simulink model "microgrid"  (R2021b)
settings: Solver=ode23tb  StartTime=0.0  StopTime=1  FixedStep=5e-6  RelTol=1e-3  EnableMultiTasking=on
PreLoadFcn:
  | % ---- microgrid : PreLoadFcn -------------------------------------
  | % Loads every base-workspace parameter this model needs.
  | %   SolarPVMPPTBoostData.mlx : PV array, boost converter, MPPT controller
  | %   microgridParams.m        : bus, battery, grid, drain, droop  (struct mg)
  | try
  |     mgDir = fileparts(which('microgrid'));
  |     if ~isempty(mgDir) && ~contains([path pathsep], [mgDir pathsep])
  |         addpath(mgDir);
  |     end
  |     evalc('SolarPVMPPTBoostData');
  |     microgridParams;
  |     clear mgDir
  |     disp('microgrid: parameters loaded (SolarPVMPPTBoostData + microgridParams).');
  | catch mgErr
  |     warning('microgrid:paramLoadFailed', ...
  |             'Could not load model parameters: %s', mgErr.message);
  |     clear mgErr
  | end
values from neighbouring files (symbols this model uses):
  mg = evalin('base','mg')    [microgridCheck.m]    (also in microgridParams.m = struct(); microgridScenario.m)
undefined symbols (not defined in the file or in its folder): boostController, dcVoltage, Ion, Lithium, sensor, solarPanel, solarPlant
libraries: powerlib_extras x46, fl_lib x12, simulink x8, nesl_utility x8, spsSeriesRLCBranchLib x7, spsCurrentMeasurementLib x7, spsGroundLib x6, spsVoltageMeasurementLib x6, spsIGBTDiodeLib x4, spsVariableResistorLib x4, slpidlib x4, ee_lib x3
(part 3 of 3)

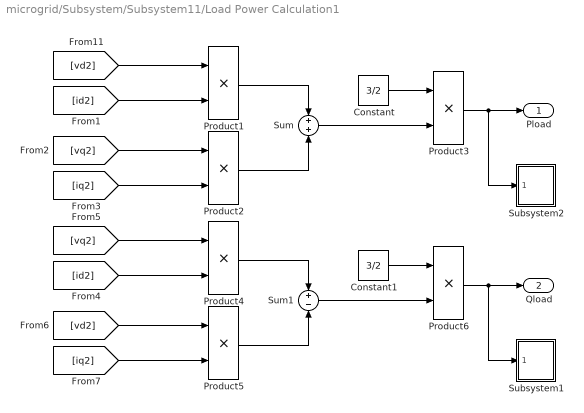
== system microgrid/Subsystem/Subsystem11/Load Power Calculation1 ==
  Constant : Constant  Value=3/2
  Constant1 : Constant  Value=3/2
  Product{1..6} (6 alike) : Product  RndMeth=Zero
  Subsystem1 : Subsystem
  Subsystem2 : Subsystem
  Sum : Sum  Inputs=+|+
  Sum1 : Sum  Inputs=+|-
  Pload : Outport
  Qload : Outport  Port=2
  wires:
  Product6/1 -> Qload/1, Subsystem1/1(Qacload)
  Constant1/1 -> Product6/1
  Sum1/1 -> Product6/2
  Product5/1 -> Sum1/2
  Product4/1 -> Sum1/1
  [iq2] -> Product5/2
  [vd2] -> Product5/1
  [id2] -> Product4/2
  [vq2] -> Product4/1
  Product3/1 -> Pload/1, Subsystem2/1(Pload)
  Constant/1 -> Product3/1
  Sum/1 -> Product3/2
  Product2/1 -> Sum/2
  Product1/1 -> Sum/1
  [iq2] -> Product2/2
  [vq2] -> Product2/1
  [id2] -> Product1/2
  [vd2] -> Product1/1

== system microgrid/Subsystem/Subsystem11/Load Power Calculation2 ==
  Constant : Constant  Value=3/2
  Constant1 : Constant  Value=3/2
  Product{1..6} (6 alike) : Product  RndMeth=Zero
  Subsystem1 : Subsystem
  Subsystem2 : Subsystem
  Sum : Sum  Inputs=+|+
  Sum1 : Sum  Inputs=+|-
  Pload : Outport
  Qload : Outport  Port=2
  wires:
  [vd3] -> Product1/1
  [id3] -> Product1/2
  [vq3] -> Product2/1
  [iq3] -> Product2/2
  Product1/1 -> Sum/1
  Product2/1 -> Sum/2
  Sum/1 -> Product3/2
  Constant/1 -> Product3/1
  Product3/1 -> Pload/1, Subsystem2/1(Pload)
  [vq3] -> Product4/1
  [id3] -> Product4/2
  [vd3] -> Product5/1
  [iq3] -> Product5/2
  Product4/1 -> Sum1/1
  Product5/1 -> Sum1/2
  Sum1/1 -> Product6/2
  Constant1/1 -> Product6/1
  Product6/1 -> Qload/1, Subsystem1/1(Qacload)

== system microgrid/PV + Boost/PV Control/Constant Voltage/Current control ==
  e : Inport
  Integrator : Integrator  LimitOutput=on  UpperSaturationLimit=1.5  LowerSaturationLimit=-1.5
  Ki : Gain  Gain=1/boostController.mppCurrentZeroTimeConst
  Kp : Gain  Gain=boostController.mppCurrentGain
  Saturation : Saturate  UpperLimit=1.5  LowerLimit=-1.5
  Sum7 : Sum  Inputs=|++
  u : Outport  VectorParamsAs1DForOutWhenUnconnected=off
  wires:
  Integrator/1 -> Sum7/2
  Saturation/1 -> u/1
  Sum7/1 -> Saturation/1
  e/1 -> Kp/1
  Kp/1 -> Ki/1, Sum7/1
  Ki/1 -> Integrator/1

== system microgrid/PV + Boost/PV Control/Constant Voltage/Voltage control ==
  e : Inport
  1/T : Gain  Gain=1/boostController.mppVoltageZeroTimeConst
  Integrator : Integrator  LimitOutput=on  UpperSaturationLimit=boostController.mppVoltageLoopMax  LowerSaturationLimit=boostController.mppVoltageLoopMin
  Kp : Gain  Gain=boostController.mppVoltageGain
  Saturation : Saturate  UpperLimit=boostController.mppVoltageLoopMax  LowerLimit=boostController.mppVoltageLoopMin
  Sum7 : Sum  Inputs=|++
  u : Outport  VectorParamsAs1DForOutWhenUnconnected=off
  wires:
  Integrator/1 -> Sum7/2
  Saturation/1 -> u/1
  Sum7/1 -> Saturation/1
  e/1 -> Kp/1
  Kp/1 -> 1/T/1, Sum7/1
  1/T/1 -> Integrator/1

== system microgrid/PV + Boost/PV Control/Maximum Power Point/MPPT ==
  Ipv : Inport
  Vpv : Inport  Port=2
  Add : Sum
  Constant1 : Constant  Value=solarPlant.voltMPPT
  Initialize : Subsystem
  MPPT Algorithm : Subsystem  Variant=on
  MPPT End Value : Constant  Value=solarPlant.endMPPTValue
  Subtract5 : Sum  Inputs=-+
  Switch : Switch  Threshold=solarPlant.endMPPTValue
  Switch5 : Switch  Criteria=u2 > Threshold  Threshold=solarPlant.startMPPTValue
  start MPPT Voltage : Constant  Value=solarPlant.startMPPTValue
  Vmpp : Outport  VectorParamsAs1DForOutWhenUnconnected=off
  tag scope: Ipvnow=global, Vdec=global, Vinc=global, Vpvnow=global
  wires:
  Switch5/1 -> Add/1, Subtract5/2
  Add/1 -> [Vinc]  "INC"
  start MPPT Voltage/1 -> Switch5/3
  Vpv/1 -> [Vpvnow], Switch5/2, Switch5/1, MPPT Algorithm/2(Vpv)
  Constant1/1 -> Add/2, Subtract5/1
  Subtract5/1 -> [Vdec]  "DEC"
  Ipv/1 -> [Ipvnow], MPPT Algorithm/1(Ipv)
  MPPT Algorithm/1(Vmpp) -> Initialize/1(In)
  Initialize/1(Out) -> Switch/3, Switch/2
  Switch/1 -> Vmpp/1
  MPPT End Value/1 -> Switch/1

== system microgrid/PV + Boost/PV Control/Maximum Power Point/MPPT Subsystem ==
  note: Current controller
  note: Voltage Control
  VpvRef : Inport
  Vpv : Inport  Port=2
  IL : Inport  Port=3
  "Vo " : Inport  Port=4
  Constant : Constant  Value=solarPlant.startMPPTValue
  Current control : Subsystem
  Divide : Product  Inputs=*/
  PWM Generator : eePwmGenerator/PWM Generator  CarrCount=Up  Tper=1/solarPlant.converterSwitchingFrequency  Tdelay=0  Ts=1/(10*solarPlant.converterSwitchingFrequency)
  Rate Transition1 : RateTransition  OutPortSampleTime=1/(10*solarPlant.converterSwitchingFrequency)
  Saturation : Saturate  UpperLimit=1  LowerLimit=0
  Subtract : Sum  Inputs=-+
  Sum : Sum  Inputs=|+-
  Sum2 : Sum  Inputs=|--
  Sum3 : Sum  Inputs=|++
  Switch : Switch  Criteria=u2 > Threshold  Threshold=dcVoltage.avgDCVoltage*0.7
  Transfer Fcn (with initial states) : simulink_extras/Additional Linear/Transfer Fcn (with initial states)  N=[1]  D=[0.00001 1]  X0=solarPlant.startMPPTValue
  Voltage control : Subsystem
  G : Outport
  wires:
  Subtract/1 -> Divide/1
  Voltage control/1(u) -> Sum2/1
  Current control/1(u) -> Sum3/1
  Sum2/1 -> Current control/1(e)
  "Vo "/1 -> Switch/2, Switch/1
  VpvRef/1 -> Transfer Fcn (with initial states)/1
  Constant/1 -> Switch/3
  Switch/1 -> Divide/2, Subtract/2
  Vpv/1 -> Subtract/1, Sum/2
  Saturation/1 -> Rate Transition1/1  "set"
  Rate Transition1/1 -> PWM Generator/1
  PWM Generator/1 -> G/1
  Divide/1 -> Sum3/2
  Sum/1 -> Voltage control/1(e)
  IL/1 -> Sum2/2
  Transfer Fcn (with initial states)/1 -> Sum/1
  Sum3/1 -> Saturation/1

== system microgrid/Subsystem/Inverter Control Measurements3/PLL/PI ==
  e : Inport
  Gain1 : Gain  Gain=10
  Gain2 : Gain  Gain=100
  Integrator : Integrator
  Saturation : Saturate  UpperLimit=inf  LowerLimit=-inf
  Sum1 : Sum  Inputs=|++
  w : Outport
  wires:
  Integrator/1 -> Sum1/2
  Gain1/1 -> Sum1/1
  e/1 -> Gain2/1, Gain1/1
  Gain2/1 -> Integrator/1
  Saturation/1 -> w/1
  Sum1/1 -> Saturation/1

== system microgrid/Subsystem/Inverter Control Measurements3/PLL/Subsystem3 ==
  wabc : Inport
  LPF vq7 : powerlib_extras/Discrete  Control Blocks/Discrete 1st-Order Filter  FilterType=Lowpass  Tc=10e-3  Ts=5e-6  Initialize=off  Vac_Init=[0.8 -25 60]  Vdc_Init=0  PlotResponse=off  param1=[1 100 0.1]
      settings: SourceProductBaseCode=PS
  To Workspace1 : ToWorkspace  VariableName=wabc_real  SampleTime=-1
  To Workspace2 : ToWorkspace  VariableName=wabc_real_fil  SampleTime=-1
  Zero-Order Hold : ZeroOrderHold  SampleTime=5e-6
  tag scope: w_abc=global
  wires:
  LPF vq7/1 -> To Workspace2/1
  wabc/1 -> Zero-Order Hold/1
  Zero-Order Hold/1 -> LPF vq7/1, To Workspace1/1, [w_abc]

== system microgrid/Subsystem/Inverter Control Measurements3/PLL/abc  - d//q ==
  abc : Inport
  tita : Inport  Port=2
  abc  - alfa/beta : Subsystem
  alfa/beta - dq : Subsystem
  d/q : Outport
  wires:
  tita/1 -> alfa/beta - dq/2(tita)
  alfa/beta - dq/1(d/q) -> d/q/1
  abc/1 -> abc  - alfa/beta/1(abc)
  abc  - alfa/beta/1(alfa/beta) -> alfa/beta - dq/1(alfa/beta)

== system microgrid/Subsystem/Subsystem11/Load Power Calculation1/Subsystem1 ==
  Qacload : Inport
  LPF vq7 : powerlib_extras/Discrete  Control Blocks/Discrete 1st-Order Filter  FilterType=Lowpass  Tc=10e-3  Ts=5e-6  Initialize=off  Vac_Init=[0.8 -25 60]  Vdc_Init=0  PlotResponse=off  param1=[1 100 0.1]
      settings: SourceProductBaseCode=PS
  To Workspace1 : ToWorkspace  VariableName=Qacload3  SampleTime=-1
  To Workspace2 : ToWorkspace  VariableName=Qacload_3  SampleTime=-1
  Zero-Order Hold : ZeroOrderHold  SampleTime=5e-6
  tag scope: Qacload3=global
  wires:
  Qacload/1 -> Zero-Order Hold/1
  Zero-Order Hold/1 -> [Qacload3], To Workspace2/1, LPF vq7/1
  LPF vq7/1 -> To Workspace1/1

== system microgrid/Subsystem/Subsystem11/Load Power Calculation1/Subsystem2 ==
  Pload : Inport
  LPF vq7 : powerlib_extras/Discrete  Control Blocks/Discrete 1st-Order Filter  FilterType=Lowpass  Tc=10e-3  Ts=5e-6  Initialize=off  Vac_Init=[0.8 -25 60]  Vdc_Init=0  PlotResponse=off  param1=[1 100 0.1]
      settings: SourceProductBaseCode=PS
  To Workspace1 : ToWorkspace  VariableName=Pacload3  SampleTime=-1
  To Workspace2 : ToWorkspace  VariableName=Pacload_3  SampleTime=-1
  Zero-Order Hold : ZeroOrderHold  SampleTime=5e-6
  tag scope: Pacload3=global
  wires:
  Pload/1 -> Zero-Order Hold/1
  Zero-Order Hold/1 -> [Pacload3], To Workspace2/1, LPF vq7/1
  LPF vq7/1 -> To Workspace1/1

== system microgrid/Subsystem/Subsystem11/Load Power Calculation2/Subsystem1 ==
  Qacload : Inport
  LPF vq7 : powerlib_extras/Discrete  Control Blocks/Discrete 1st-Order Filter  FilterType=Lowpass  Tc=10e-3  Ts=5e-6  Initialize=off  Vac_Init=[0.8 -25 60]  Vdc_Init=0  PlotResponse=off  param1=[1 100 0.1]
      settings: SourceProductBaseCode=PS
  To Workspace1 : ToWorkspace  VariableName=Qacload2  SampleTime=-1
  To Workspace2 : ToWorkspace  VariableName=Qacload_2  SampleTime=-1
  Zero-Order Hold : ZeroOrderHold  SampleTime=5e-6
  tag scope: Qacload2=global
  wires:
  Qacload/1 -> Zero-Order Hold/1
  Zero-Order Hold/1 -> [Qacload2], To Workspace2/1, LPF vq7/1
  LPF vq7/1 -> To Workspace1/1

== system microgrid/Subsystem/Subsystem11/Load Power Calculation2/Subsystem2 ==
  Pload : Inport
  LPF vq7 : powerlib_extras/Discrete  Control Blocks/Discrete 1st-Order Filter  FilterType=Lowpass  Tc=10e-3  Ts=5e-6  Initialize=off  Vac_Init=[0.8 -25 60]  Vdc_Init=0  PlotResponse=off  param1=[1 100 0.1]
      settings: SourceProductBaseCode=PS
  To Workspace1 : ToWorkspace  VariableName=Pacload2  SampleTime=-1
  To Workspace2 : ToWorkspace  VariableName=Pacload_2  SampleTime=-1
  Zero-Order Hold : ZeroOrderHold  SampleTime=5e-6
  tag scope: Pacload2=global
  wires:
  Pload/1 -> Zero-Order Hold/1
  Zero-Order Hold/1 -> [Pacload2], To Workspace2/1, LPF vq7/1
  LPF vq7/1 -> To Workspace1/1

== system microgrid/PV + Boost/PV Control/Maximum Power Point/MPPT/Initialize ==
  In : Inport
  Constant : Constant  Value=solarPlant.startMPPTValue
  Constant2 : Constant
  Integrator : Integrator
  Switch1 : Switch  Criteria=u2 > Threshold  Threshold=solarPlant.startMPPTValue
  Switch2 : Switch  Criteria=u2 > Threshold  Threshold=solarPlant.timeMPPT
  Out : Outport
  wires:
  Constant/1 -> Switch1/3
  Switch1/1 -> Switch2/1
  In/1 -> Switch1/2, Switch1/1
  Switch2/1 -> Out/1
  Constant2/1 -> Integrator/1
  [Vpvnow] -> Switch2/3
  Integrator/1 -> Switch2/2

== system microgrid/PV + Boost/PV Control/Maximum Power Point/MPPT/MPPT Algorithm ==
  Ipv : Inport
  Vpv : Inport  Port=2
  IncrementalConductance : Subsystem  VariantControl=incrementalConductance
  PerturbationAndObsrvation : Subsystem  VariantControl=perturbationAndObservation
  Vmpp : Outport  VectorParamsAs1DForOutWhenUnconnected=off

== system microgrid/PV + Boost/PV Control/Maximum Power Point/MPPT Subsystem/Current control ==
  e : Inport
  Integrator : Integrator  InitialCondition=1  LimitOutput=on  UpperSaturationLimit=1  LowerSaturationLimit=-0.5
  Ki : Gain  Gain=1/boostController.mppCurrentZeroTimeConst
  Kp : Gain  Gain=boostController.mppCurrentGain
  Saturation : Saturate  UpperLimit=1  LowerLimit=-0.3
  Sum7 : Sum  Inputs=|++
  u : Outport  VectorParamsAs1DForOutWhenUnconnected=off
  wires:
  Integrator/1 -> Sum7/2
  Saturation/1 -> u/1
  Sum7/1 -> Saturation/1
  e/1 -> Kp/1
  Kp/1 -> Ki/1, Sum7/1
  Ki/1 -> Integrator/1

== system microgrid/PV + Boost/PV Control/Maximum Power Point/MPPT Subsystem/Voltage control ==
  e : Inport
  1/T : Gain  Gain=1/boostController.mppVoltageZeroTimeConst
  Integrator : Integrator  LimitOutput=on  UpperSaturationLimit=boostController.mppVoltageLoopMax  LowerSaturationLimit=boostController.mppVoltageLoopMin
  Kp : Gain  Gain=boostController.mppVoltageGain
  Saturation : Saturate  UpperLimit=boostController.mppVoltageLoopMax  LowerLimit=boostController.mppVoltageLoopMin
  Sum7 : Sum  Inputs=|++
  u : Outport  VectorParamsAs1DForOutWhenUnconnected=off
  wires:
  Integrator/1 -> Sum7/2
  Saturation/1 -> u/1
  Sum7/1 -> Saturation/1
  e/1 -> Kp/1
  Kp/1 -> 1/T/1, Sum7/1
  1/T/1 -> Integrator/1

== system microgrid/Subsystem/Inverter Control Measurements3/PLL/abc  - d//q/abc  - alfa//beta ==
  abc : Inport
  Mux : Mux  Inputs=2
  d_s : Fcn  Expr=(-1/sqrt(3)*u[2])+(1/sqrt(3)*u[3])
  q_s : Fcn  Expr=(2/3)*u[1]-(1/3)*u[2]-(1/3)*u[3]
  alfa/beta : Outport
  wires:
  abc/1 -> q_s/1, d_s/1
  d_s/1 -> Mux/1
  q_s/1 -> Mux/2
  Mux/1 -> alfa/beta/1

== system microgrid/Subsystem/Inverter Control Measurements3/PLL/abc  - d//q/alfa//beta - dq ==
  alfa/beta : Inport
  tita : Inport  Port=2
  Mux : Mux  Inputs=2
  Mux1 : Mux  Inputs=2
  d : Fcn  Expr=u[2]*sin(u[3]) + u[1]*cos(u[3])
  q : Fcn  Expr=-u[1]*sin(u[3]) + u[2]*cos(u[3])
  d/q : Outport
  wires:
  d/1 -> Mux/1
  q/1 -> Mux/2
  Mux/1 -> d/q/1
  alfa/beta/1 -> Mux1/1
  tita/1 -> Mux1/2
  Mux1/1 -> d/1, q/1

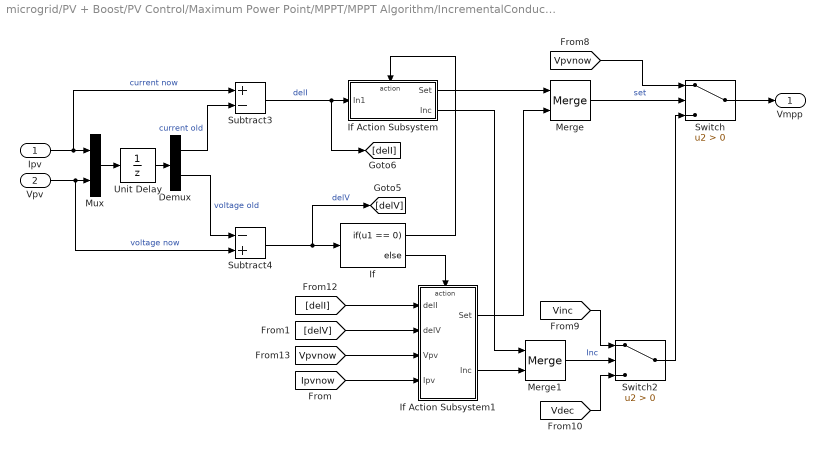
== system microgrid/PV + Boost/PV Control/Maximum Power Point/MPPT/MPPT Algorithm/IncrementalConductance ==
  Ipv : Inport
  Vpv : Inport  Port=2
  Demux : Demux  Outputs=2
  If : If  IfExpression=u1 == 0
  If Action Subsystem : Subsystem  TreatAsAtomicUnit=on
  If Action Subsystem1 : Subsystem  TreatAsAtomicUnit=on
  Merge : Merge
  Merge1 : Merge
  Mux : Mux  Inputs=2
  Subtract3 : Sum  Inputs=+-
  Subtract4 : Sum  Inputs=-+
  Switch : Switch  Criteria=u2 > Threshold
  Switch2 : Switch  Criteria=u2 > Threshold
  Unit Delay : UnitDelay  InitialCondition=solarPlant.startMPPTValue  SampleTime=solarPlant.timeMPPT  HasFrameUpgradeWarning=on
  Vmpp : Outport  VectorParamsAs1DForOutWhenUnconnected=off
  wires:
  Merge1/1 -> Switch2/2  "Inc"
  [Vpvnow] -> Switch/1
  If Action Subsystem1/2(Inc) -> Merge1/2
  If Action Subsystem/2(Inc) -> Merge1/1
  If/2 -> If Action Subsystem1/Action
  If Action Subsystem/1(Set) -> Merge/1
  [delV] -> If Action Subsystem1/2(delV)
  [delI] -> If Action Subsystem1/1(delI)
  Merge/1 -> Switch/2  "set"
  If Action Subsystem1/1(Set) -> Merge/2
  If/1 -> If Action Subsystem/Action
  [Vpvnow] -> If Action Subsystem1/3(Vpv)
  Switch2/1 -> Switch/3
  [Ipvnow] -> If Action Subsystem1/4(Ipv)
  Ipv/1 -> Mux/1, Subtract3/1  "current now"
  Unit Delay/1 -> Demux/1
  Mux/1 -> Unit Delay/1
  Vpv/1 -> Subtract4/2, Mux/2  "voltage now"
  Demux/2 -> Subtract4/1  "voltage old"
  Demux/1 -> Subtract3/2  "current old"
  Subtract3/1 -> [delI], If Action Subsystem/1(In1)  "delI"
  Subtract4/1 -> [delV], If/1  "delV"
  Switch/1 -> Vmpp/1
  [Vdec] -> Switch2/3
  [Vinc] -> Switch2/1

== system microgrid/PV + Boost/PV Control/Maximum Power Point/MPPT/MPPT Algorithm/PerturbationAndObsrvation ==
  note: Both voltage and power is in falling trend
  note: Both voltage and power is in raising trend
  Ipv : Inport
  Vpv : Inport  Port=2
  AND : Logic  IconShape=distinctive  AllPortsSameDT=off  OutDataTypeStr=boolean
  Compare To Constant : simulink/Logic and Bit Operations/Compare To Constant  relop=>=  const=0  OutDataTypeStr=boolean
  Compare To Zero1 : simulink/Logic and Bit Operations/Compare To Zero  relop=>=  OutDataTypeStr=boolean
  Demux : Demux  Outputs=2
  Mux : Mux  Inputs=2
  NOR : Logic  Operator=NOR  IconShape=distinctive  AllPortsSameDT=off  OutDataTypeStr=boolean
  OR : Logic  Operator=OR  IconShape=distinctive  AllPortsSameDT=off  OutDataTypeStr=boolean
  Product : Product
  Product1 : Product
  Subtract : Sum  Inputs=+-
  Subtract4 : Sum  Inputs=-+
  Switch4 : Switch  Criteria=u2 ~= 0
  Unit Delay : UnitDelay  InitialCondition=solarPlant.startMPPTValue  SampleTime=solarPlant.timeMPPT  HasFrameUpgradeWarning=on
  Zero-Order Hold : ZeroOrderHold  SampleTime=solarPlant.timeMPPT
  Vmpp : Outport  VectorParamsAs1DForOutWhenUnconnected=off
  wires:
  NOR/1 -> OR/2
  OR/1 -> Switch4/2
  Compare To Zero1/1 -> AND/2, NOR/2
  AND/1 -> OR/1
  Compare To Constant/1 -> AND/1, NOR/1
  Mux/1 -> Unit Delay/1
  Ipv/1 -> Product1/2, Mux/1
  Demux/1 -> Product/1
  Unit Delay/1 -> Demux/1
  Demux/2 -> Product/2, Subtract4/1  "voltage old"
  Vpv/1 -> Product1/1, Subtract4/2, Mux/2  "voltage now"
  Product1/1 -> Subtract/1  "power now"
  Product/1 -> Subtract/2  "power old"
  Subtract4/1 -> Compare To Zero1/1  "delV"
  Subtract/1 -> Compare To Constant/1  "delPower"
  Switch4/1 -> Zero-Order Hold/1
  [Vdec] -> Switch4/3
  [Vinc] -> Switch4/1
  Zero-Order Hold/1 -> Vmpp/1

== system microgrid/PV + Boost/PV Control/Maximum Power Point/MPPT/MPPT Algorithm/IncrementalConductance/If Action Subsystem ==
  In1 : Inport
  Action Port : ActionPort  ActionPortLabel=if(u1 == 0)
  Compare To Constant : simulink/Logic and Bit Operations/Compare To Constant  relop===  const=0  OutDataTypeStr=boolean
  Compare To Zero2 : simulink/Logic and Bit Operations/Compare To Zero  relop=>  OutDataTypeStr=boolean
  Set : Outport  VectorParamsAs1DForOutWhenUnconnected=off
  Inc : Outport  Port=2  VectorParamsAs1DForOutWhenUnconnected=off
  wires:
  Compare To Constant/1 -> Set/1  "Yes"
  Compare To Zero2/1 -> Inc/1  "Yes"
  In1/1 -> Compare To Zero2/1, Compare To Constant/1  "delI"

== system microgrid/PV + Boost/PV Control/Maximum Power Point/MPPT/MPPT Algorithm/IncrementalConductance/If Action Subsystem1 ==
  delI : Inport
  delV : Inport  Port=2
  Vpv : Inport  Port=3
  Ipv : Inport  Port=4
  Action Port : ActionPort  ActionPortLabel=else
  Add : Sum
  Compare To Zero : simulink/Logic and Bit Operations/Compare To Zero  relop===  OutDataTypeStr=boolean
  Compare To Zero1 : simulink/Logic and Bit Operations/Compare To Zero  relop=>  OutDataTypeStr=boolean
  Divide : Product  Inputs=*/
  Product : Product
  Set : Outport  VectorParamsAs1DForOutWhenUnconnected=off
  Inc : Outport  Port=2  VectorParamsAs1DForOutWhenUnconnected=off
  wires:
  delI/1 -> Divide/1
  delV/1 -> Divide/2
  Divide/1 -> Product/1
  Add/1 -> Compare To Zero1/1, Compare To Zero/1
  Compare To Zero/1 -> Set/1  "set"
  Vpv/1 -> Product/2
  Product/1 -> Add/1
  Ipv/1 -> Add/2
  Compare To Zero1/1 -> Inc/1  "Increase"
